simulink model "c_CollectAdmis"  (R2024b)
settings: Solver=VariableStepAuto  StartTime=0.0  StopTime=10.0  RelTol=1e-3
values from neighbouring files (symbols this model uses):
  Mim0 = 0+0.001    (= 0.001)    [InitISM_AII.m]
  Tamb = 300    [InitISM_AII.m]
undefined symbols (not defined in the file or in its folder): DebitAirEvt, DebitMoteurEvt, ManifoldMassTest, ManifoldPressureTest, ManifoldTemperatureTest, ManifoldTimeTest, P0, TempsEvt
settings Model: Creator=a030141  LastModifiedBy=ramse
settings DebuggingCC: UnderspecifiedInitializationDetection=Classic  MergeDetectMultiDrivingBlocksExec=none
settings ModelReferenceCC: PropagateSignalLabelsOutOfModel=off

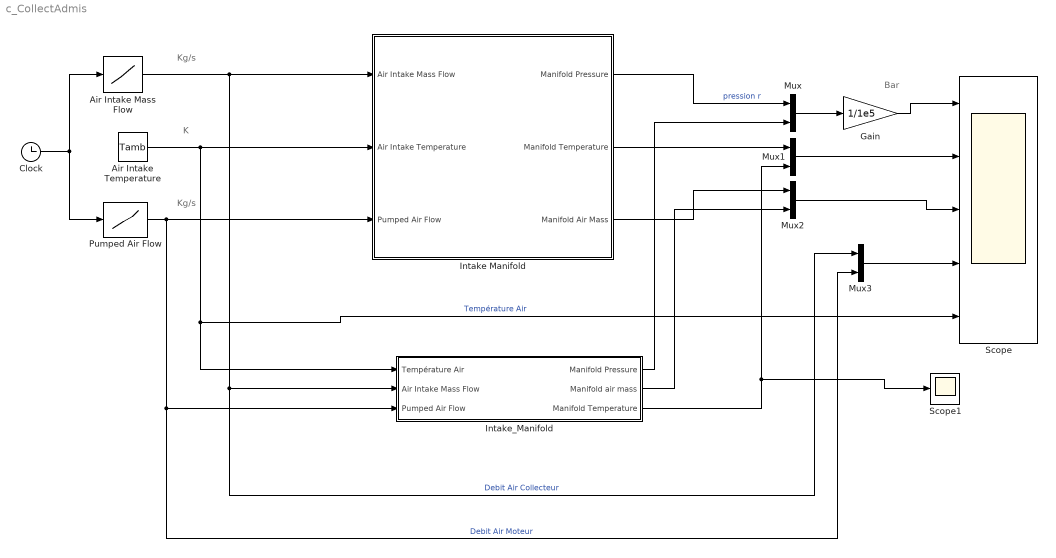
== system c_CollectAdmis ==
  note: Kg/s
  note: Kg/s
  note: K
  note: Bar
  Air Intake Mass Flow : Lookup  InputValues=TempsEvt  Table=DebitAirEvt
  Air Intake Temperature : Constant  Value=Tamb
  Clock : Clock
  Gain : Gain  Gain=1/1e5  SaturateOnIntegerOverflow=on  OutDataTypeStr=Inherit: Same as input  ParamDataTypeStr=Inherit: Same as input
  Intake Manifold : Subsystem
  Intake_Manifold : Subsystem
  Mux{,1..3} (4 alike) : Mux  Inputs=2
  Pumped Air Flow : Lookup  InputValues=TempsEvt  Table=DebitMoteurEvt
  Scope : Scope  NumInputPorts=5
  Scope1 : Scope
  wires:
  Clock/1 -> Pumped Air Flow/1, Air Intake Mass Flow/1
  Air Intake Mass Flow/1 -> Mux3/1, Intake_Manifold/2(Air Intake Mass Flow), Intake Manifold/1(Air Intake Mass Flow)  "Debit Air Collecteur"
  Pumped Air Flow/1 -> Mux3/2, Intake_Manifold/3(Pumped Air Flow), Intake Manifold/3(Pumped Air Flow)  "Debit Air Moteur"
  Air Intake Temperature/1 -> Intake_Manifold/1(Température Air), Scope/5, Intake Manifold/2(Air Intake Temperature)  "Température Air"
  Mux/1 -> Gain/1
  Gain/1 -> Scope/1
  Mux1/1 -> Scope/2
  Mux2/1 -> Scope/3
  Mux3/1 -> Scope/4
  Intake Manifold/1(Manifold Pressure) -> Mux/1  "pression r"
  Intake Manifold/3(Manifold Air Mass) -> Mux2/1
  Intake Manifold/2(Manifold Temperature) -> Mux1/1
  Intake_Manifold/3(Manifold Temperature) -> Scope1/1, Mux1/2
  Intake_Manifold/1(Manifold Pressure) -> Mux/2
  Intake_Manifold/2(Manifold air mass) -> Mux2/2

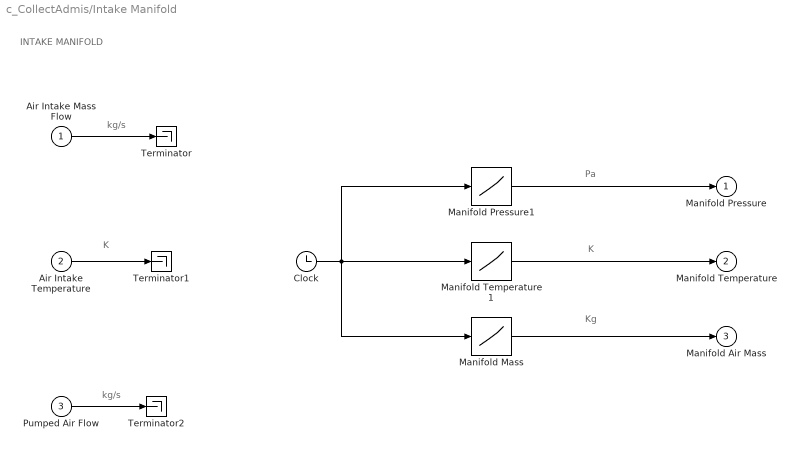
== system c_CollectAdmis/Intake Manifold ==
  note: INTAKE MANIFOLD
  note: kg/s
  note: K
  note: kg/s
  note: Kg
  note: K
  note: Pa
  Air Intake Mass Flow : Inport
  Air Intake Temperature : Inport  Port=2
  Pumped Air Flow : Inport  Port=3
  Clock : Clock
  Manifold Mass : Lookup  InputValues=ManifoldTimeTest  Table=ManifoldMassTest
  Manifold Pressure1 : Lookup  InputValues=ManifoldTimeTest  Table=ManifoldPressureTest
  Manifold Temperature1 : Lookup  InputValues=ManifoldTimeTest  Table=ManifoldTemperatureTest
  Terminator : Terminator
  Terminator1 : Terminator
  Terminator2 : Terminator
  Manifold Pressure : Outport
  Manifold Temperature : Outport  Port=2
  Manifold Air Mass : Outport  Port=3
  wires:
  Pumped Air Flow/1 -> Terminator2/1
  Air Intake Mass Flow/1 -> Terminator/1
  Air Intake Temperature/1 -> Terminator1/1
  Manifold Pressure1/1 -> Manifold Pressure/1
  Manifold Temperature1/1 -> Manifold Temperature/1
  Manifold Mass/1 -> Manifold Air Mass/1
  Clock/1 -> Manifold Temperature1/1, Manifold Pressure1/1, Manifold Mass/1

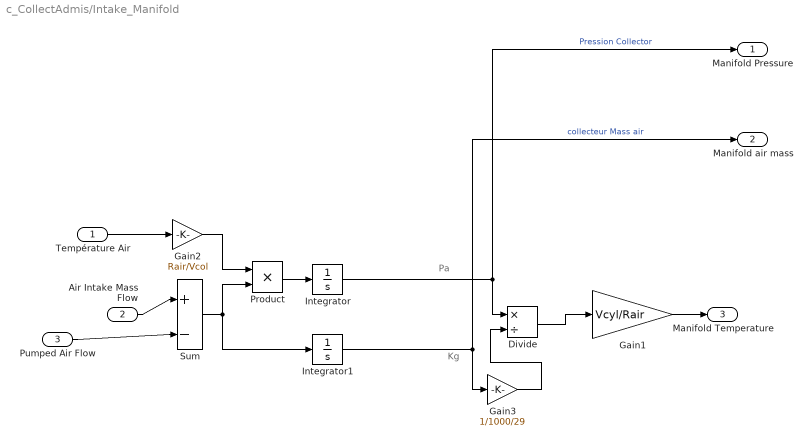
== system c_CollectAdmis/Intake_Manifold ==
  note: Kg
  note: Pa
  Température Air : Inport
  Air Intake Mass Flow : Inport  Port=2
  Pumped Air Flow : Inport  Port=3
  Divide : Product  Inputs=*/
  Gain1 : Gain  Gain=Vcyl/Rair
  Gain2 : Gain  Gain=Rair/Vcol
  Gain3 : Gain  Gain=1/1000/29
  Integrator : Integrator  InitialCondition=P0
  Integrator1 : Integrator  InitialCondition=Mim0
  Product : Product
  Sum : Sum  Inputs=|+-
  Manifold Pressure : Outport
  Manifold air mass : Outport  Port=2
  Manifold Temperature : Outport  Port=3
  wires:
  Sum/1 -> Integrator1/1, Product/2
  Gain2/1 -> Product/1
  Product/1 -> Integrator/1
  Gain1/1 -> Manifold Temperature/1
  Integrator/1 -> Manifold Pressure/1, Divide/1  "Pression Collector"
  Integrator1/1 -> Manifold air mass/1, Gain3/1  "collecteur Mass air"
  Gain3/1 -> Divide/2
  Divide/1 -> Gain1/1
  Air Intake Mass Flow/1 -> Sum/1
  Température Air/1 -> Gain2/1
  Pumped Air Flow/1 -> Sum/2
